simulink model "singlearealfc"  (R2025a)
settings: Solver=VariableStepAuto  StartTime=0.0  StopTime=50  RelTol=1e-3
settings Model: Creator=Lijoofficial  LastModifiedBy=Lijoofficial

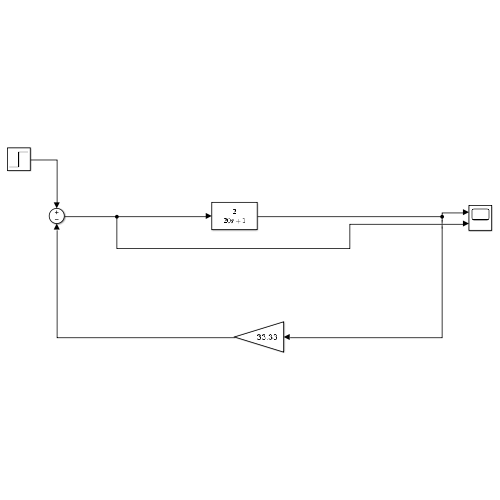
[thumbnail: Simulink's stored preview of the top-level diagram]
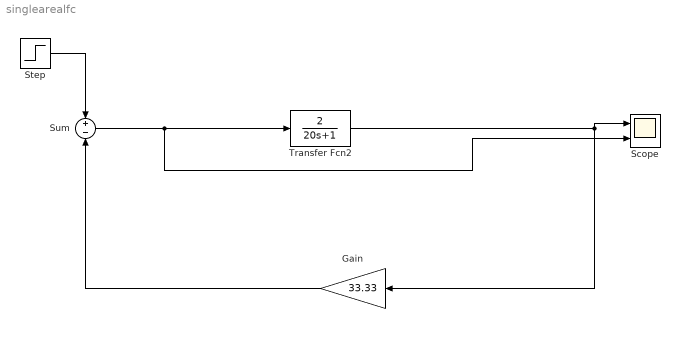
== system singlearealfc ==
  Gain : Gain  Gain=33.33
  Scope : Scope  NumInputPorts=2
      settings: ActiveDisplayYMinimum=-0.0036946506283985865  ActiveDisplayYMaximum=0.03325185565558729
  Step : Step  SampleTime=0
  Sum : Sum  Inputs=+-
  Transfer Fcn2 : TransferFcn  Numerator=2  Denominator=[20 1]
  wires:
  Gain/1 -> Sum/2
  Transfer Fcn2/1 -> Gain/1, Scope/1
  Step/1 -> Sum/1
  Sum/1 -> Scope/2, Transfer Fcn2/1
